simulink model "LETS_GOOOOOO"  (R2020b)
settings: Solver=VariableStepAuto  StartTime=0.0  StopTime=60  RelTol=1e-3
values from neighbouring files (symbols this model uses):
  A_2 = zeros(3)    [MPC_tune.m]
  B_2 = I_inv    [MPC_tune.m]
  C_2 = eye(3)    [MPC_tune.m]
  D_2 = zeros(3)    [MPC_tune.m]
  I_inv = inv(I_mat)    [MPC_tune.m]
  m = 941.102    [Linear_tuning.m]
  TcgCatia = [1 0 0 ... (first row only)    [MPC_tune.m]
undefined symbols (not defined in the file or in its folder): A_kal, B_kal, C_kal, Continuous, D_kal, delta_time, F_tot_max, Fb1_l, Fb1_u, Fb2_l, Fb2_u, Fb3_l, Fb3_u, Fb4_l, Fb4_u, Fc1_l, Fc1_u, Fc2_l, Fc2_u, Fc3_l, Fc3_u, fprop, Ft1_l, Ft1_u, Ft2_l, Ft2_u, Ft3_l, Ft3_u, Ft4_l, Ft4_u, g, r_0, r_cgCatia, r_trajectory, rho, T, t_finalgust, theta0, time, Time, time_delay, Tzy_Shard, u0_final, u0_ini, u1_final, u1_ini, u2_final, u2_ini, u_0, u_1, u_2, v_0, ZI_Cx, ZI_Cy, ZI_Cz, ZI_p, ZI_q, ZI_r
libraries: dspsigops x11, simulink x6, pid_lib x6, fuzblock x3, sharedutil x1, mpclib x1, dspmathops x1, ctrlSharedLib x1
(part 2 of 2)

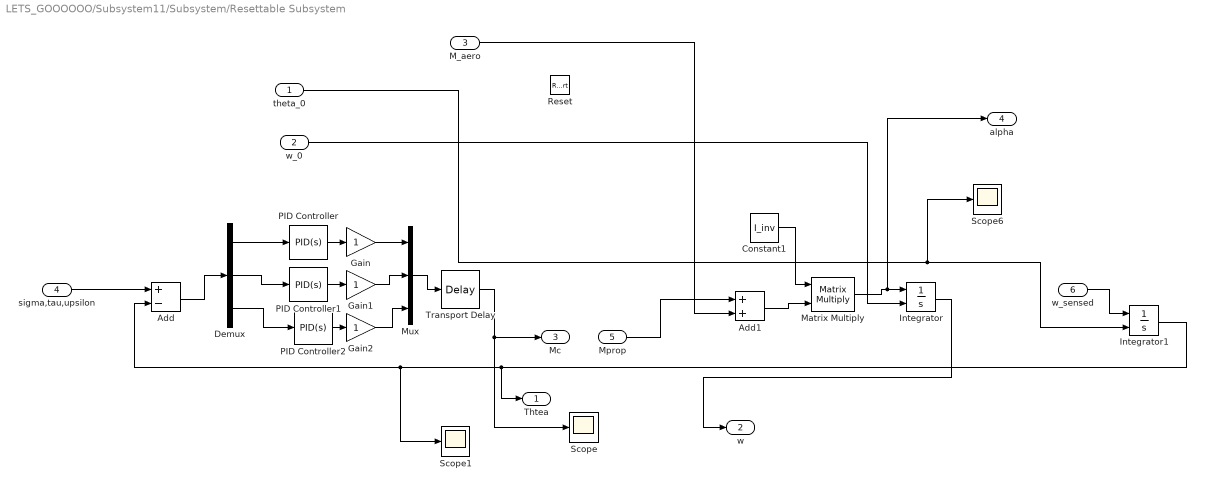
== system LETS_GOOOOOO/Subsystem11/Subsystem/Resettable Subsystem ==
  theta_0 : Inport
  w_0 : Inport  Port=2
  M_aero : Inport  Port=3
  sigma,tau,upsilon : Inport  Port=4
  Mprop : Inport  Port=5
  w_sensed : Inport  Port=6
  Reset : ResetPort  DisableCoverage=on  ResetTriggerType=either
  Add : Sum  Inputs=+-
  Add1 : Sum
  Constant1 : Constant  Value=I_inv
  Demux : Demux  Outputs=3
  Gain : Gain
  Gain1 : Gain
  Gain2 : Gain
  Integrator : Integrator  InitialConditionSource=external  InitialCondition=[0.15;-0.2;0.01]
  Integrator1 : Integrator  InitialConditionSource=external  InitialCondition=[0.01;-0.01;0.005]
  Matrix Multiply : Product  Multiplication=Matrix(*)
  Mux : Mux  Inputs=3
  PID Controller : pid_lib/PID Controller  Controller=PID  Form=Parallel  TimeDomain=Continuous-time  UseExternalTs=off  SampleTime=-1  IntegratorMethod=Forward Euler  FilterMethod=Forward Euler  ControllerParametersSource=internal  P=76.4274415550338  I=3.57793373088927  D=400.875615235633  UseFilter=on  N=5.45397025421619  TunerSelectOption=Transfer Function Based (PID Tuner App)  InitialConditionSource=internal  InitialConditionForIntegrator=0  InitialConditionForFilter=0  DifferentiatorICPrevScaledInput=0  ExternalReset=none  TrackingMode=off  Kt=1  LimitOutput=off  SatLimitsSource=internal  UpperSaturationLimit=inf  LowerSaturationLimit=-inf  LinearizeAsGain=on  AntiWindupMode=none  Kb=1  POutMin=[]  POutMax=[]  IOutMin=[]  IOutMax=[]  DOutMin=[]  DOutMax=[]  NOutMin=[]  NOutMax=[]  SumOutMin=[]  SumOutMax=[]  SaturationOutMin=[]  SaturationOutMax=[]  PParamMin=[]  PParamMax=[]  IParamMin=[]  IParamMax=[]  DParamMin=[]  DParamMax=[]  NParamMin=[]  NParamMax=[]  KbParamMin=[]  KbParamMax=[]  KtParamMin=[]  KtParamMax=[]  KbOutMin=[]  KbOutMax=[]  KtOutMin=[]  KtOutMax=[]  IntegratorOutMin=[]  IntegratorOutMax=[]  FilterOutMin=[]  FilterOutMax=[]  SumI1OutMin=[]  SumI1OutMax=[]  SumI2OutMin=[]  SumI2OutMax=[]  SumI3OutMin=[]  SumI3OutMax=[]  SumI4OutMin=[]  SumI4OutMax=[]  SumDOutMin=[]  SumDOutMax=[]  DifferentiatorOutMin=[]  DifferentiatorOutMax=[]  FilterDiffOutCoefMin=[]  FilterDiffOutCoefMax=[]  ReciprocalOutMin=[]  ReciprocalOutMax=[]  SumDenOutMin=[]  SumDenOutMax=[]  SumNumOutMin=[]  SumNumOutMax=[]  DivideOutMin=[]  DivideOutMax=[]  UdiffTsProdOutMin=[]  UdiffTsProdOutMax=[]  NTsProdOutMin=[]  NTsProdOutMax=[]  UintegralTsProdOutMin=[]  UintegralTsProdOutMax=[]  UngainTsProdOutMin=[]  UngainTsProdOutMax=[]  IntegratorContinuousStateAttributes=''  IntegratorStateMustResolveToSignalObject=off  IntegratorRTWStateStorageClass=Auto  FilterContinuousStateAttributes=''  FilterStateMustResolveToSignalObject=off  FilterRTWStateStorageClass=Auto  ParallelPVariant=InternalParameters  IdealPVariant=Disabled  IVariant=InternalParameters  DVariant=InternalParameters  IntegratorVariant=Continuous  SatVariant=Disabled  AWVariant=Passthrough  PCopyVariant=Disabled  TRVariant=Disabled  FdbkBlocksVariant=Forward  IdealPFdbkVariant=Disabled  SatFdbkVariant=Disabled  DerivativeFilterVariant=ContFilter  NVariant=InternalParameters  NCopyVariant=Disabled  FilterICVariant=InternalICsFilter  IntegratorICVariant=InternalICs  ExternalResetVariant=Disabled  TRSumVariant=Passthrough  SumFdbkVariant=Disabled  SumVariant=Sum_PID  TsampFilterVariant=InternalTs  TsampNgainVariant=Passthrough  TsampIntegralVariant=Passthrough  ExternalSaturationOutDataTypeStr=Inherit: Same as second input
  PID Controller1 : pid_lib/PID Controller  Controller=PID  Form=Parallel  TimeDomain=Continuous-time  UseExternalTs=off  SampleTime=-1  IntegratorMethod=Forward Euler  FilterMethod=Forward Euler  ControllerParametersSource=internal  P=-202.527799620363  I=-9.48129403471772  D=-1062.29457146841  UseFilter=on  N=5.45397025421619  TunerSelectOption=Transfer Function Based (PID Tuner App)  InitialConditionSource=internal  InitialConditionForIntegrator=0  InitialConditionForFilter=0  DifferentiatorICPrevScaledInput=0  ExternalReset=none  TrackingMode=off  Kt=1  LimitOutput=off  SatLimitsSource=internal  UpperSaturationLimit=inf  LowerSaturationLimit=-inf  LinearizeAsGain=on  AntiWindupMode=none  Kb=1  POutMin=[]  POutMax=[]  IOutMin=[]  IOutMax=[]  DOutMin=[]  DOutMax=[]  NOutMin=[]  NOutMax=[]  SumOutMin=[]  SumOutMax=[]  SaturationOutMin=[]  SaturationOutMax=[]  PParamMin=[]  PParamMax=[]  IParamMin=[]  IParamMax=[]  DParamMin=[]  DParamMax=[]  NParamMin=[]  NParamMax=[]  KbParamMin=[]  KbParamMax=[]  KtParamMin=[]  KtParamMax=[]  KbOutMin=[]  KbOutMax=[]  KtOutMin=[]  KtOutMax=[]  IntegratorOutMin=[]  IntegratorOutMax=[]  FilterOutMin=[]  FilterOutMax=[]  SumI1OutMin=[]  SumI1OutMax=[]  SumI2OutMin=[]  SumI2OutMax=[]  SumI3OutMin=[]  SumI3OutMax=[]  SumI4OutMin=[]  SumI4OutMax=[]  SumDOutMin=[]  SumDOutMax=[]  DifferentiatorOutMin=[]  DifferentiatorOutMax=[]  FilterDiffOutCoefMin=[]  FilterDiffOutCoefMax=[]  ReciprocalOutMin=[]  ReciprocalOutMax=[]  SumDenOutMin=[]  SumDenOutMax=[]  SumNumOutMin=[]  SumNumOutMax=[]  DivideOutMin=[]  DivideOutMax=[]  UdiffTsProdOutMin=[]  UdiffTsProdOutMax=[]  NTsProdOutMin=[]  NTsProdOutMax=[]  UintegralTsProdOutMin=[]  UintegralTsProdOutMax=[]  UngainTsProdOutMin=[]  UngainTsProdOutMax=[]  IntegratorContinuousStateAttributes=''  IntegratorStateMustResolveToSignalObject=off  IntegratorRTWStateStorageClass=Auto  FilterContinuousStateAttributes=''  FilterStateMustResolveToSignalObject=off  FilterRTWStateStorageClass=Auto  ParallelPVariant=InternalParameters  IdealPVariant=Disabled  IVariant=InternalParameters  DVariant=InternalParameters  IntegratorVariant=Continuous  SatVariant=Disabled  AWVariant=Passthrough  PCopyVariant=Disabled  TRVariant=Disabled  FdbkBlocksVariant=Forward  IdealPFdbkVariant=Disabled  SatFdbkVariant=Disabled  DerivativeFilterVariant=ContFilter  NVariant=InternalParameters  NCopyVariant=Disabled  FilterICVariant=InternalICsFilter  IntegratorICVariant=InternalICs  ExternalResetVariant=Disabled  TRSumVariant=Passthrough  SumFdbkVariant=Disabled  SumVariant=Sum_PID  TsampFilterVariant=InternalTs  TsampNgainVariant=Passthrough  TsampIntegralVariant=Passthrough  ExternalSaturationOutDataTypeStr=Inherit: Same as second input
  PID Controller2 : pid_lib/PID Controller  Controller=PID  Form=Parallel  TimeDomain=Continuous-time  UseExternalTs=off  SampleTime=-1  IntegratorMethod=Forward Euler  FilterMethod=Forward Euler  ControllerParametersSource=internal  P=-232.294042315359  I=-10.8747940867059  D=-1218.42384402842  UseFilter=on  N=5.45397025421619  TunerSelectOption=Transfer Function Based (PID Tuner App)  InitialConditionSource=internal  InitialConditionForIntegrator=0  InitialConditionForFilter=0  DifferentiatorICPrevScaledInput=0  ExternalReset=none  TrackingMode=off  Kt=1  LimitOutput=off  SatLimitsSource=internal  UpperSaturationLimit=inf  LowerSaturationLimit=-inf  LinearizeAsGain=on  AntiWindupMode=none  Kb=1  POutMin=[]  POutMax=[]  IOutMin=[]  IOutMax=[]  DOutMin=[]  DOutMax=[]  NOutMin=[]  NOutMax=[]  SumOutMin=[]  SumOutMax=[]  SaturationOutMin=[]  SaturationOutMax=[]  PParamMin=[]  PParamMax=[]  IParamMin=[]  IParamMax=[]  DParamMin=[]  DParamMax=[]  NParamMin=[]  NParamMax=[]  KbParamMin=[]  KbParamMax=[]  KtParamMin=[]  KtParamMax=[]  KbOutMin=[]  KbOutMax=[]  KtOutMin=[]  KtOutMax=[]  IntegratorOutMin=[]  IntegratorOutMax=[]  FilterOutMin=[]  FilterOutMax=[]  SumI1OutMin=[]  SumI1OutMax=[]  SumI2OutMin=[]  SumI2OutMax=[]  SumI3OutMin=[]  SumI3OutMax=[]  SumI4OutMin=[]  SumI4OutMax=[]  SumDOutMin=[]  SumDOutMax=[]  DifferentiatorOutMin=[]  DifferentiatorOutMax=[]  FilterDiffOutCoefMin=[]  FilterDiffOutCoefMax=[]  ReciprocalOutMin=[]  ReciprocalOutMax=[]  SumDenOutMin=[]  SumDenOutMax=[]  SumNumOutMin=[]  SumNumOutMax=[]  DivideOutMin=[]  DivideOutMax=[]  UdiffTsProdOutMin=[]  UdiffTsProdOutMax=[]  NTsProdOutMin=[]  NTsProdOutMax=[]  UintegralTsProdOutMin=[]  UintegralTsProdOutMax=[]  UngainTsProdOutMin=[]  UngainTsProdOutMax=[]  IntegratorContinuousStateAttributes=''  IntegratorStateMustResolveToSignalObject=off  IntegratorRTWStateStorageClass=Auto  FilterContinuousStateAttributes=''  FilterStateMustResolveToSignalObject=off  FilterRTWStateStorageClass=Auto  ParallelPVariant=InternalParameters  IdealPVariant=Disabled  IVariant=InternalParameters  DVariant=InternalParameters  IntegratorVariant=Continuous  SatVariant=Disabled  AWVariant=Passthrough  PCopyVariant=Disabled  TRVariant=Disabled  FdbkBlocksVariant=Forward  IdealPFdbkVariant=Disabled  SatFdbkVariant=Disabled  DerivativeFilterVariant=ContFilter  NVariant=InternalParameters  NCopyVariant=Disabled  FilterICVariant=InternalICsFilter  IntegratorICVariant=InternalICs  ExternalResetVariant=Disabled  TRSumVariant=Passthrough  SumFdbkVariant=Disabled  SumVariant=Sum_PID  TsampFilterVariant=InternalTs  TsampNgainVariant=Passthrough  TsampIntegralVariant=Passthrough  ExternalSaturationOutDataTypeStr=Inherit: Same as second input
  Scope : Scope
  Scope1 : Scope
  Scope6 : Scope
  Transport Delay : TransportDelay  DelayTime=0.1
  Thtea : Outport
  w : Outport  Port=2
  Mc : Outport  Port=3
  alpha : Outport  Port=4
  wires:
  Transport Delay/1 -> Mc/1, Scope/1
  Constant1/1 -> Matrix Multiply/1
  PID Controller2/1 -> Gain2/1
  PID Controller/1 -> Gain/1
  Matrix Multiply/1 -> alpha/1, Integrator/1
  Demux/3 -> PID Controller2/1
  Mux/1 -> Transport Delay/1
  sigma,tau,upsilon/1 -> Add/1
  Gain/1 -> Mux/1
  w_0/1 -> Integrator/2
  Gain2/1 -> Mux/3
  Add/1 -> Demux/1
  Add1/1 -> Matrix Multiply/2
  PID Controller1/1 -> Gain1/1
  Integrator/1 -> w/1
  theta_0/1 -> Integrator1/2, Scope6/1
  Demux/2 -> PID Controller1/1
  Gain1/1 -> Mux/2
  M_aero/1 -> Add1/2
  Demux/1 -> PID Controller/1
  Integrator1/1 -> Thtea/1, Scope1/1, Add/2
  Mprop/1 -> Add1/1
  w_sensed/1 -> Integrator1/1

== system LETS_GOOOOOO/Subsystem11/Subsystem/Resettable Subsystem1 ==
  sigma,tau,upsilon : Inport
  Maero : Inport  Port=2
  w0 : Inport  Port=3
  theta0 : Inport  Port=4
  reset : Inport  Port=5
  Mprop : Inport  Port=6
  wsensed : Inport  Port=7
  Add : Sum  Inputs=-+
  Subsystem : Subsystem
  error : Outport
  theta : Outport  Port=2
  w : Outport  Port=3
  Mc : Outport  Port=4
  alpha : Outport  Port=5
  wires:
  theta0/1 -> Subsystem/4(tehat0)
  Subsystem/2(w) -> w/1
  Add/1 -> error/1
  Maero/1 -> Subsystem/1(M_aero)
  sigma,tau,upsilon/1 -> Add/2, Subsystem/2(sigma,tau,upsilon)  "sigma, tau, upsilon"
  Subsystem/1(theta) -> Add/1, theta/1
  w0/1 -> Subsystem/3(w0)
  reset/1 -> Subsystem/5(reset)
  Subsystem/3(Mc) -> Mc/1
  Mprop/1 -> Subsystem/6(Mprop)
  Subsystem/4(alpha) -> alpha/1
  wsensed/1 -> Subsystem/7(wsensed)

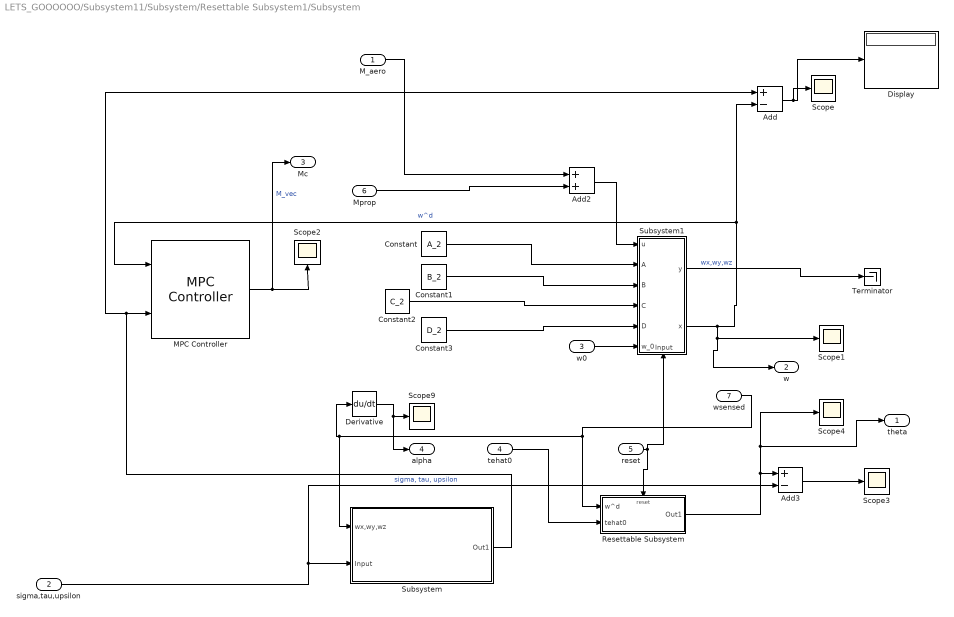
== system LETS_GOOOOOO/Subsystem11/Subsystem/Resettable Subsystem1/Subsystem ==
  M_aero : Inport
  sigma,tau,upsilon : Inport  Port=2
  w0 : Inport  Port=3
  tehat0 : Inport  Port=4
  reset : Inport  Port=5
  Mprop : Inport  Port=6
  wsensed : Inport  Port=7
  Add : Sum  Inputs=+-
  Add2 : Sum
  Add3 : Sum  Inputs=+-
  Constant : Constant  Value=A_2
  Constant1 : Constant  Value=B_2
  Constant2 : Constant  Value=C_2
  Constant3 : Constant  Value=D_2
  Derivative : Derivative
  Display : Display
  MPC Controller : mpclib/MPC Controller  SCDEnableBlockLinearizationSpecification=on  mpcobj=MPCDesignerSession.AppData.Controllers.MPC  is_multiple=0  enable_value=0  return_u0=off  updateMPCinCallerWorkspace=on  md_inport=off  mv_inport=off  uref_inport=off  return_cost=off  return_mvseq=off  return_qpstatus=off  return_xseq=off  return_state=off  return_ovseq=off  state_inport=off  umin_inport=off  umax_inport=off  ymin_inport=off  ymax_inport=off  cc_inport=off  ywt_inport=off  uwt_inport=off  duwt_inport=off  rhoeps_inport=off  pm_inport=off  MaximumP=10  HorizonChoice=FixedHorizon  n_ts=0.1  n_p=10  n_mv=3  n_md=0  n_ud=0  n_mo=3  n_uo=0  BlockDataType=double  SampleTimeInherited=off  switch_inport=off
  Resettable Subsystem : Subsystem  TreatAsAtomicUnit=on
  Scope{,1..4,9} (6 alike) : Scope
  Subsystem : Subsystem
  Subsystem1 : Subsystem
      settings: PortSchema="{\"entries\":[{\"content\":{\"sides\":[{\"content\":{\"connectorIds\":[\"In1\",\"In2\",\"In3\",\"In4\",\"In5\",\"In6\"]},\"type\":\"ConnectorPlacement.EquallySpacedRectSide\",\"uuid\":\"7d9460a7-3adf-4f89-91e7-b456f7078c86\"},{\"content\":{\"connectorIds\":[\"Out1\",\"Out2\"],\"side\":\"RIGHT\"},\"type\":\"ConnectorPlacement.EquallySpacedRectSide\",\"uuid\":\"f1bf29ac-ed67-4ce4-91e2-85f2b90efa08\"},{\"content\":{\"connectorIds\":[],\"side\":\"TOP\"},\"type\":\"ConnectorPlacement.EquallySpacedRectSide\",\"uuid\":\"d922c634-a6d8-424b-a167-3b858780e5fe\"},{\"content\":{\"connectorIds\":[\"In7\"],\"side\":\"BOTTOM\"},\"type\":\"ConnectorPlacement.EquallySpacedRectSide\",\"uuid\":\"f177f641-1570-409d-a38e-cef2b78f705f\"},{\"content\":{\"connectorIds\":[],\"side\":\"HIDDEN\"},\"type\":\"ConnectorPlacement.EquallySpacedRectSide\",\"uuid\":\"30cf80c6-7b26-40df-a778-919a6a544dd2\"}]},\"type\":\"ConnectorPlacement.EquallySpacedConnector\",\"uuid\":\"27252b95-3211-4624-87a6-4be9d32d6c6a\"}],\"packageUris\":[\"http://schema.mathworks.com/mf0/Connector/R2020b\"],\"version\":\"1.0\"}"
  Terminator : Terminator
  theta : Outport
  w : Outport  Port=2
  Mc : Outport  Port=3
  alpha : Outport  Port=4
  wires:
  Subsystem1/1(y) -> Terminator/1  "wx,wy,wz"
  Derivative/1 -> alpha/1, Scope9/1
  Resettable Subsystem/1(Out1) -> Scope4/1, theta/1, Add3/1
  Add/1 -> Display/1, Scope/1
  Add3/1 -> Scope3/1
  Add2/1 -> Subsystem1/1(u)
  sigma,tau,upsilon/1 -> Add3/2, Subsystem/2(Input)  "sigma, tau, upsilon"
  Subsystem/1(Out1) -> Add/1, MPC Controller/2
  M_aero/1 -> Add2/1
  Constant2/1 -> Subsystem1/4(C)
  Constant3/1 -> Subsystem1/5(D)
  Subsystem1/2(x) -> Add/2, MPC Controller/1, w/1, Scope1/1  "w^d"
  MPC Controller/1 -> Mc/1, Scope2/1  "M_vec"
  Constant/1 -> Subsystem1/2(A)
  Constant1/1 -> Subsystem1/3(B)
  w0/1 -> Subsystem1/6(w_0)
  tehat0/1 -> Resettable Subsystem/2(tehat0)
  reset/1 -> Subsystem1/7(Input), Resettable Subsystem/Reset
  Mprop/1 -> Add2/2
  wsensed/1 -> Resettable Subsystem/1(w^d), Subsystem/1(wx,wy,wz), Derivative/1

== system LETS_GOOOOOO/Subsystem11/Subsystem/Resettable Subsystem1/Subsystem/Resettable Subsystem ==
  w^d : Inport
  tehat0 : Inport  Port=2
  Reset : ResetPort  DisableCoverage=on
  Integrator : Integrator  InitialConditionSource=external  InitialCondition=theta0
  Scope : Scope
  Out1 : Outport
  wires:
  tehat0/1 -> Integrator/2
  w^d/1 -> Integrator/1
  Integrator/1 -> Scope/1, Out1/1

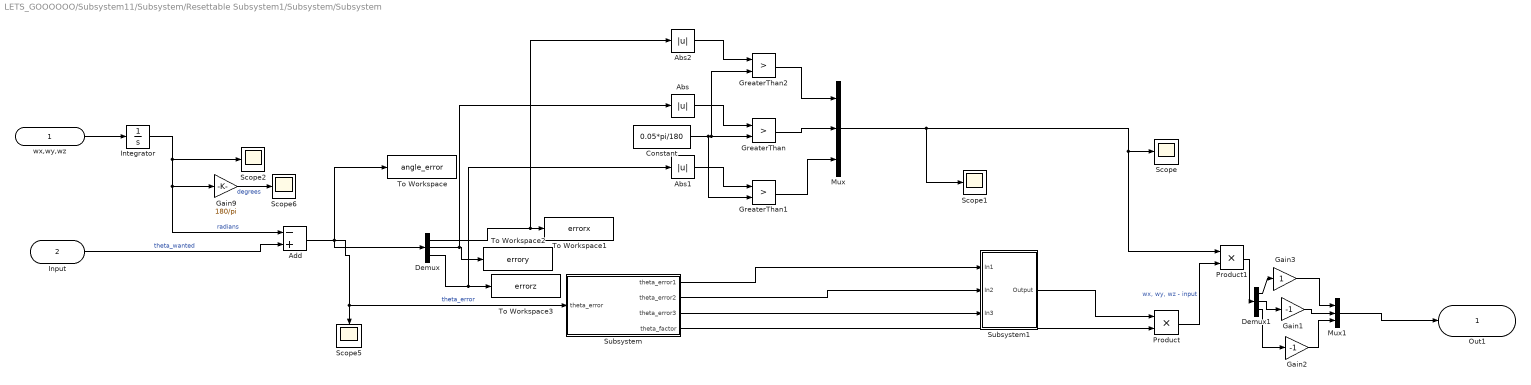
== system LETS_GOOOOOO/Subsystem11/Subsystem/Resettable Subsystem1/Subsystem/Subsystem ==
  wx,wy,wz : Inport
  Input : Inport  Port=2
  Abs : Abs
  Abs1 : Abs
  Abs2 : Abs
  Add : Sum  Inputs=-+
  Constant : Constant  Value=0.05*pi/180
  Demux : Demux  Outputs=3
  Demux1 : Demux  Outputs=3
  Gain1 : Gain  Gain=-1
  Gain2 : Gain  Gain=-1
  Gain3 : Gain
  Gain9 : Gain  Gain=180/pi
  GreaterThan : RelationalOperator  Operator=>  OutDataTypeStr=boolean  RndMeth=Simplest
  GreaterThan1 : RelationalOperator  Operator=>  OutDataTypeStr=boolean  RndMeth=Simplest
  GreaterThan2 : RelationalOperator  Operator=>  OutDataTypeStr=boolean  RndMeth=Simplest
  Integrator : Integrator  InitialCondition=[0;0;0]
  Mux : Mux  Inputs=3
  Mux1 : Mux  Inputs=3
  Product : Product
  Product1 : Product
  Scope{,1..2,5..6} (5 alike) : Scope
  Subsystem : Subsystem
  Subsystem1 : Subsystem
  To Workspace : ToWorkspace  VariableName=angle_error  SampleTime=-1
  To Workspace1 : ToWorkspace  VariableName=errorx  SaveFormat=Timeseries  SampleTime=-1
      settings: Save2DSignal=2-D array (concatenate along first dimension)
  To Workspace2 : ToWorkspace  VariableName=errory  SaveFormat=Timeseries  SampleTime=-1
  To Workspace3 : ToWorkspace  VariableName=errorz  SaveFormat=Timeseries  SampleTime=-1
  Out1 : Outport
  wires:
  Integrator/1 -> Add/1, Gain9/1, Scope2/1  "radians"
  Add/1 -> To Workspace/1, Demux/1, Subsystem/1(theta_error), Scope5/1  "theta_error"
  Gain9/1 -> Scope6/1  "degrees"
  Input/1 -> Add/2  "theta_wanted"
  Product/1 -> Product1/2  "wx, wy, wz - input"
  wx,wy,wz/1 -> Integrator/1
  Subsystem/4(theta_factor) -> Product/2
  Demux/2 -> Abs/1, To Workspace2/1
  Demux/3 -> Abs1/1, To Workspace3/1
  Demux/1 -> Abs2/1, To Workspace1/1
  Subsystem/1(theta_error1) -> Subsystem1/1(In1)
  Subsystem/2(theta_error2) -> Subsystem1/2(In2)
  Subsystem/3(theta_error3) -> Subsystem1/3(In3)
  Subsystem1/1(Output) -> Product/1
  Abs/1 -> GreaterThan/1
  Constant/1 -> GreaterThan1/2, GreaterThan2/2, GreaterThan/2
  Abs1/1 -> GreaterThan1/1
  Abs2/1 -> GreaterThan2/1
  GreaterThan2/1 -> Mux/1
  GreaterThan/1 -> Mux/2
  GreaterThan1/1 -> Mux/3
  Mux/1 -> Scope1/1, Scope/1, Product1/1
  Product1/1 -> Demux1/1
  Mux1/1 -> Out1/1
  Demux1/2 -> Gain1/1
  Demux1/3 -> Gain2/1
  Demux1/1 -> Gain3/1
  Gain3/1 -> Mux1/1
  Gain1/1 -> Mux1/2
  Gain2/1 -> Mux1/3

== system LETS_GOOOOOO/Subsystem11/Subsystem/Resettable Subsystem1/Subsystem/Subsystem1 ==
  u : Inport
  A : Inport  Port=2
  B : Inport  Port=3
  C : Inport  Port=4
  D : Inport  Port=5
  w_0 : Inport  Port=6
  Input : Inport  Port=7
  Product{,1..3} (4 alike) : Product  SCDEnableBlockLinearizationSpecification=on  Multiplication=Matrix(*)
  Resettable Subsystem : Subsystem  TreatAsAtomicUnit=on
  Sum : Sum  Inputs=|++
  Sum1 : Sum  Inputs=++|
  dxTerm : Terminator
  y : Outport  VectorParamsAs1DForOutWhenUnconnected=off
  x : Outport  Port=2  VectorParamsAs1DForOutWhenUnconnected=off
  wires:
  Sum/1 -> Resettable Subsystem/1(alpha), dxTerm/1  "dx"
  Product3/1 -> Sum1/1  "Cx"
  Product/1 -> Sum/1  "Bu"
  u/1 -> Product2/2, Product/2
  Product2/1 -> Sum1/2  "Du"
  Resettable Subsystem/1(x) -> x/1, Product1/2, Product3/2  "x"
  A/1 -> Product1/1
  Product1/1 -> Sum/2  "Ax"
  C/1 -> Product3/1
  B/1 -> Product/1
  D/1 -> Product2/1
  Sum1/1 -> y/1
  w_0/1 -> Resettable Subsystem/2(omega0)
  Input/1 -> Resettable Subsystem/Reset

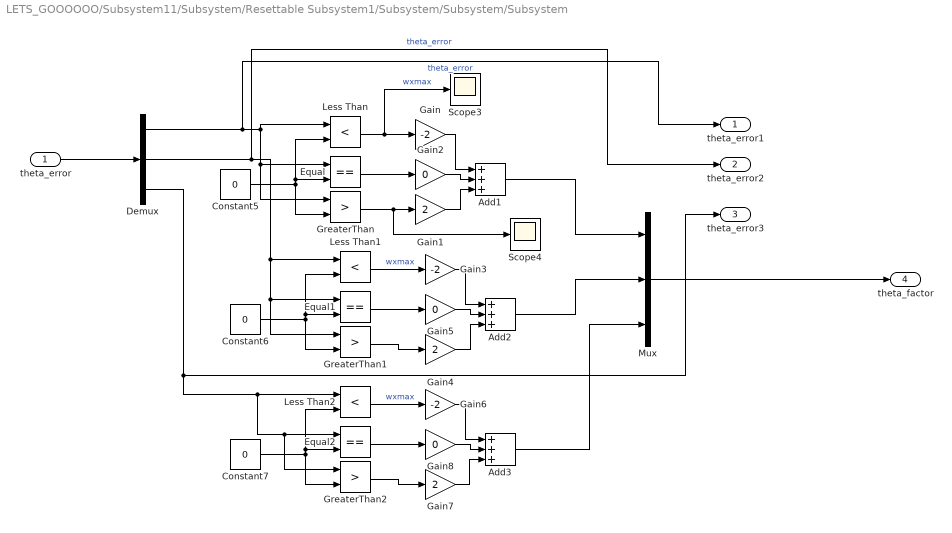
== system LETS_GOOOOOO/Subsystem11/Subsystem/Resettable Subsystem1/Subsystem/Subsystem/Subsystem ==
  theta_error : Inport
  Add1 : Sum  Inputs=+++
  Add2 : Sum  Inputs=+++
  Add3 : Sum  Inputs=+++
  Constant5 : Constant  Value=0
  Constant6 : Constant  Value=0
  Constant7 : Constant  Value=0
  Demux : Demux  Outputs=3
  Equal : RelationalOperator  Operator===  OutDataTypeStr=boolean  RndMeth=Simplest
  Equal1 : RelationalOperator  Operator===  OutDataTypeStr=boolean  RndMeth=Simplest
  Equal2 : RelationalOperator  Operator===  OutDataTypeStr=boolean  RndMeth=Simplest
  Gain : Gain  Gain=-2
  Gain1 : Gain  Gain=2
  Gain2 : Gain  Gain=0
  Gain3 : Gain  Gain=-2
  Gain4 : Gain  Gain=2
  Gain5 : Gain  Gain=0
  Gain6 : Gain  Gain=-2
  Gain7 : Gain  Gain=2
  Gain8 : Gain  Gain=0
  GreaterThan : RelationalOperator  Operator=>  OutDataTypeStr=boolean  RndMeth=Simplest
  GreaterThan1 : RelationalOperator  Operator=>  OutDataTypeStr=boolean  RndMeth=Simplest
  GreaterThan2 : RelationalOperator  Operator=>  OutDataTypeStr=boolean  RndMeth=Simplest
  Less Than : RelationalOperator  Operator=<  OutDataTypeStr=boolean  RndMeth=Simplest
  Less Than1 : RelationalOperator  Operator=<  OutDataTypeStr=boolean  RndMeth=Simplest
  Less Than2 : RelationalOperator  Operator=<  OutDataTypeStr=boolean  RndMeth=Simplest
  Mux : Mux  Inputs=3
  Scope3 : Scope
  Scope4 : Scope
  theta_error1 : Outport
  theta_error2 : Outport  Port=2
  theta_error3 : Outport  Port=3
  theta_factor : Outport  Port=4
  wires:
  Add1/1 -> Mux/1
  Constant5/1 -> Equal/2, Less Than/2, GreaterThan/2
  Equal2/1 -> Gain8/1
  Demux/1 -> theta_error1/1, GreaterThan/1, Equal/1, Less Than/1  "theta_error"
  GreaterThan2/1 -> Gain7/1
  Gain1/1 -> Add1/3
  Gain7/1 -> Add3/3
  Less Than1/1 -> Gain3/1  "wxmax"
  Gain6/1 -> Add3/1
  Equal/1 -> Gain2/1
  Gain5/1 -> Add2/2
  Add3/1 -> Mux/3
  GreaterThan/1 -> Scope4/1, Gain1/1
  Constant6/1 -> Equal1/2, Less Than1/2, GreaterThan1/2
  Demux/3 -> theta_error3/1, GreaterThan2/1, Equal2/1, Less Than2/1
  Gain3/1 -> Add2/1
  Constant7/1 -> Equal2/2, Less Than2/2, GreaterThan2/2
  Equal1/1 -> Gain5/1
  Gain8/1 -> Add3/2
  Gain4/1 -> Add2/3
  GreaterThan1/1 -> Gain4/1
  Gain/1 -> Add1/1
  Demux/2 -> theta_error2/1, GreaterThan1/1, Equal1/1, Less Than1/1  "theta_error"
  Gain2/1 -> Add1/2
  Add2/1 -> Mux/2
  Less Than/1 -> Scope3/1, Gain/1  "wxmax"
  Less Than2/1 -> Gain6/1  "wxmax"
  theta_error/1 -> Demux/1
  Mux/1 -> theta_factor/1

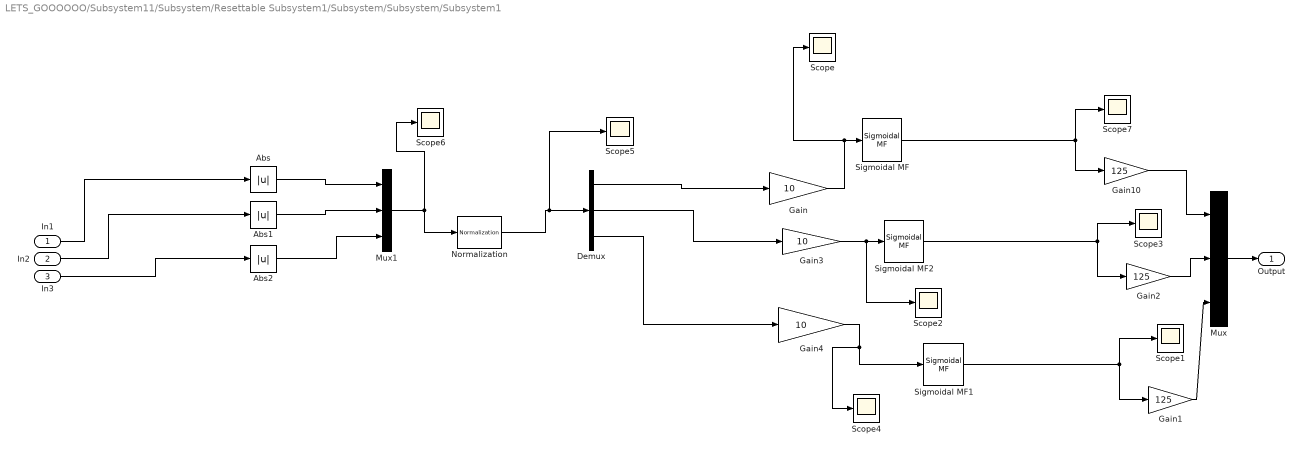
== system LETS_GOOOOOO/Subsystem11/Subsystem/Resettable Subsystem1/Subsystem/Subsystem/Subsystem1 ==
  In1 : Inport
  In2 : Inport  Port=2
  In3 : Inport  Port=3
  Abs : Abs
  Abs1 : Abs
  Abs2 : Abs
  Demux : Demux  Outputs=3
  Gain : Gain  Gain=10
  Gain1 : Gain  Gain=125
  Gain10 : Gain  Gain=125
  Gain2 : Gain  Gain=125
  Gain3 : Gain  Gain=10
  Gain4 : Gain  Gain=10
  Mux : Mux  Inputs=3
  Mux1 : Mux  Inputs=3
  Normalization : dspmathops/Normalization  NormType=Squared 2-norm  Bias=1e-10  NormOver=Each column  Dimension=1  roundingMode=Floor  overflowMode=off  accumDataTypeStr=Inherit: Same as product output  accumLastDataTypeStr=Inherit: Same as product output  outputDataTypeStr=Inherit: Same as product output  outputMin=[]  outputMax=[]  outputLastDataTypeStr=Inherit: Same as product output
  Scope{,1..7} (8 alike) : Scope
  Sigmoidal MF : fuzblock/Membership  Functions/Sigmoidal MF  a=10^(-8)  c=1000
      settings: SourceProductBaseCode=FL
  Sigmoidal MF1 : fuzblock/Membership  Functions/Sigmoidal MF  a=10^(-8)  c=1000
      settings: SourceProductBaseCode=FL
  Sigmoidal MF2 : fuzblock/Membership  Functions/Sigmoidal MF  a=10^(-8)  c=1000
      settings: SourceProductBaseCode=FL
  Output : Outport
  wires:
  Gain2/1 -> Mux/2
  Gain10/1 -> Mux/1
  Sigmoidal MF1/1 -> Gain1/1, Scope1/1
  Sigmoidal MF/1 -> Gain10/1, Scope7/1
  Sigmoidal MF2/1 -> Gain2/1, Scope3/1
  Gain/1 -> Scope/1, Sigmoidal MF/1
  Gain1/1 -> Mux/3
  Gain3/1 -> Scope2/1, Sigmoidal MF2/1
  In2/1 -> Abs1/1
  In1/1 -> Abs/1
  In3/1 -> Abs2/1
  Mux/1 -> Output/1
  Abs/1 -> Mux1/1
  Abs1/1 -> Mux1/2
  Gain4/1 -> Scope4/1, Sigmoidal MF1/1
  Abs2/1 -> Mux1/3
  Demux/3 -> Gain4/1
  Demux/1 -> Gain/1
  Demux/2 -> Gain3/1
  Mux1/1 -> Normalization/1, Scope6/1
  Normalization/1 -> Scope5/1, Demux/1

== system LETS_GOOOOOO/Subsystem11/Subsystem/Resettable Subsystem1/Subsystem/Subsystem1/Resettable Subsystem ==
  alpha : Inport
  omega0 : Inport  Port=2
  Reset : ResetPort  DisableCoverage=on
  Integrator : Integrator  InitialConditionSource=external  InitialCondition=theta0
  Scope : Scope
  x : Outport
  wires:
  omega0/1 -> Integrator/2
  alpha/1 -> Integrator/1
  Integrator/1 -> Scope/1, x/1

== matlab function LETS_GOOOOOO/Subsystem5/Subsystem/MATLAB Function6 ==
  data: F_y input; F_c1 output; M_x input; M_z input; F_c2 output; F_c3 output
function [F_c1, F_c2, F_c3] = fcn(F_y, M_x, M_z)
%CATIA trans
TcgCatia = [1 0 0;
    0 -1 0;
    0 0 -1];

%Propeller arms - changed due to CATIA errors
c_1 = [-640.1998; 0; 506.566]*10^(-3);      %Control Back Top
c_2 = [-1040.1998; 0; -493.434]*10^(-3);    %Control Back Bottom
c_3 = [2259.8002; 0; -293.434]*10^(-3);     %Control Front

%Propeller arms - rotated
c_1 = TcgCatia*c_1;
c1 = transpose(c_1);
c_2 = TcgCatia*c_2;
c2 = transpose(c_2);
c_3 = TcgCatia*c_3;
c3 = transpose(c_3);

xc_1 = c1(1);
zc_1 = c1(3);

xc_2 = c2(1);
zc_2 = c2(3);

xc_3 = c3(1);
zc_3 = c3(3);

A_control = [1 1 1;
    zc_1 zc_2 zc_3;
    xc_1 xc_2 xc_3];
A_cinv = inv(A_control);
force_control = [F_y; M_x; M_z];
controlvec = A_cinv*force_control;
F_c1 = controlvec(1);
F_c2 = controlvec(2);
F_c3 = controlvec(3);
end

== matlab function LETS_GOOOOOO/Subsystem5/MATLAB Function4 ==
  data: F1 input; F_t1 output; F2 input; F3 input; F_t2 output; F_t3 output; F_t4 output; F_b1 output; F_b2 output; F_b3 output; F_b4 output
function [F_t1, F_t2, F_t3, F_t4, F_b1, F_b2, F_b3, F_b4] = fcn(F1, F2, F3)
%F3 is one prop
%F1 is two props
%F2 is two props
F_t1 = F1/2;
F_t2 = F_t1;
F_t3 = F3;
F_t4 = F_t3;
F_b3 = F_t3;
F_b4 = F_t3;
F_b1 = F2/2;
F_b2 = F_b1;

Ft = [F_t1, F_t2, F_t3, F_t4];
Fb = [F_b1, F_b2, F_b3, F_b4];
end

== matlab function LETS_GOOOOOO/Subsystem5/Subsystem3/MATLAB Function7 ==
  data: F1 input; F_z output; F2 input; M_y output; F3 input
function [F_z, M_y] = fcn(F1, F2, F3)
xt_1 = 1.2598;
xb_1 = 2.2598;
xt_3 = -1.3402;
x_t1 = xt_1;
x_b1 = xb_1;
x_t3 = xt_3;

M_y = -100;
F_z = 0;

A_mat = [1 1;
    xt_1 xb_1];

A_inv = inv(A_mat);

force = [F1; F2];

back = A_mat*force;
backtrack = [4*F3; 4*F3*xt_3];
forceback = back+backtrack;
F_z = forceback(1);
M_y = forceback(2) + 0.15;
end

== matlab function LETS_GOOOOOO/Subsystem5/Subsystem3/MATLAB Function8 ==
  data: F_c1 input; F_y output; M_x output; F_c2 input; F_c3 input; M_z output
function [F_y, M_x, M_z] = fcn(F_c1, F_c2, F_c3)

%CATIA trans
TcgCatia = [1 0 0;
    0 -1 0;
    0 0 -1];

%Propeller arms - changed due to CATIA errors
c_1 = [-640.1998; 0; 506.566]*10^(-3);      %Control Back Top
c_2 = [-1040.1998; 0; -493.434]*10^(-3);    %Control Back Bottom
c_3 = [2259.8002; 0; -293.434]*10^(-3);     %Control Front

%Propeller arms - rotated
c_1 = TcgCatia*c_1;
c1 = transpose(c_1);
c_2 = TcgCatia*c_2;
c2 = transpose(c_2);
c_3 = TcgCatia*c_3;
c3 = transpose(c_3);

xc_1 = c1(1);
zc_1 = c1(3);

xc_2 = c2(1);
zc_2 = c2(3);

xc_3 = c3(1);
zc_3 = c3(3);


Control_forces = [F_c1; F_c2; F_c3];

A_control = [1 1 1;
        zc_1 zc_2 zc_3;
        xc_1 xc_2 xc_3]; 
Control_vec_2 = A_control*Control_forces;
F_y = Control_vec_2(1);
M_x = Control_vec_2(2);
M_z = Control_vec_2(3);
end

== matlab function LETS_GOOOOOO/Subsystem5/Subsystem3/MATLAB Function9 ==
  data: Ft1 input; F1 output; Ft2 input; F2 output; F3 output; Ft3 input; Ft4 input; Fb1 input; Fb2 input; Fb3 input; Fb4 input
function [F1, F2, F3] = fcn(Ft1, Ft2, Ft3, Ft4, Fb1, Fb2, Fb3, Fb4)
%F3 is one prop
%F1 is two props
%F2 is two props
F1 = 2*Ft1;
F2 = 2*Fb1;
F3 = Ft3;
end

== matlab function LETS_GOOOOOO/Subsystem4/MATLAB Function2 ==
  data: theta_x input; Transformation_Mat output; theta_y input; theta_z input
function Transformation_Mat  = Euler(theta_x, theta_y, theta_z)

a = cos(theta_x)*cos(theta_z);
b = cos(theta_x)*sin(theta_z);
c = - sin(theta_x);
d = sin(theta_y)*sin(theta_x)*cos(theta_z) - cos(theta_y)*sin(theta_z);
e = sin(theta_y)*sin(theta_x)*sin(theta_z) + cos(theta_y)*cos(theta_z);
f = sin(theta_y)*cos(theta_x);
g = cos(theta_y)*sin(theta_x)*cos(theta_z) + sin(theta_y)*sin(theta_z);
h = cos(theta_y)*sin(theta_x)*sin(theta_z) - sin(theta_y)*cos(theta_z);
i = cos(theta_y)*cos(theta_x);

Transformation_Mat = [a b c;
    d e f;
    g h i];


end

== matlab function LETS_GOOOOOO/Subsystem9/GPS Model ==
  settings: updateMethod=DISCRETE
  data: position input; newposition output
function newposition  = gps(position)

    % Input: position
    % Output: position with gps accuracies inclduded
    mu = 0; 
    sigma = 0.015;

    r1 = normrnd(mu, sigma);
    r2 = normrnd(mu, sigma);
    r3 = normrnd(mu, sigma);

    newposition = [0,0,0];

    newposition(1) = position(1) + r1;
    newposition(2) = position(2) + r2;
    newposition(3) = position(3) + r3;

end

== matlab function LETS_GOOOOOO/Subsystem4/MATLAB Function3 ==
  data: theta_x input; Transformation_Mat output; theta_y input; theta_z input
function Transformation_Mat  = Euler(theta_x, theta_y, theta_z)

a = cos(theta_x)*cos(theta_z);
b = cos(theta_x)*sin(theta_z);
c = - sin(theta_x);
d = sin(theta_y)*sin(theta_x)*cos(theta_z) - cos(theta_y)*sin(theta_z);
e = sin(theta_y)*sin(theta_x)*sin(theta_z) + cos(theta_y)*cos(theta_z);
f = sin(theta_y)*cos(theta_x);
g = cos(theta_y)*sin(theta_x)*cos(theta_z) + sin(theta_y)*sin(theta_z);
h = cos(theta_y)*sin(theta_x)*sin(theta_z) - sin(theta_y)*cos(theta_z);
i = cos(theta_y)*cos(theta_x);

Transformation_Mat = [a b c;
    d e f;
    g h i];


end

== matlab function LETS_GOOOOOO/Subsystem5/Subsystem/MATLAB Function ==
  data: My input; Ft1 output; Fz input; Ft2 output; Ft3 output; Ft4 output; Fb1 output; Fb2 output; Fb3 output; Fb4 output
function [Ft1, Ft2, Ft3, Ft4, Fb1, Fb2, Fb3, Fb4] = fixingpropulsionsmess(My, Fz)
xt_1 = 1.2598;
xb_1 = 2.2598;
xt_3 = -1.3402;
xb_3 = -1.3402;
x_t1 = xt_1;
x_b1 = xb_1;
x_t3 = xt_3;
x_b3 = xb_3;;

%alpha_1 = (-2*xt_1*(1/((xt_1/xb_1)-1))*(2 - (2*xb_3/xb_1)) - 4*xb_3)^2;
%alpha_2 = ((1/((xt_1/xb_1)-1))*(2-(2*xb_3/xb_1)))^2;
%alpha = alpha_1 + alpha_2;

%beta_1 = 2*My*((1/(2*xb_1))*(1 - (xt_1/xb_1)*(1/((xt_1/xb_1) -1))));
%beta_2 = 2*My*(1/((xt_1/xb_1) -1))*(1/(2*xb_1))*(1/((xt_1/xb_1) -1))*(2 - ((2*xb_3)/x_b1));
%beta_3 = 2*Fz*(1/(2*xb_1)*xt_1*(1/(xt_1/xb_1 -1)));
%beta_4 = 2*Fz*(-1/2*(1/(xt_1/xb_1 -1))*(1/(xt_1/xb_1 -1))*(2-2*xb_3/xb_1));
%beta = beta_1 + beta_2 + beta_3 + beta_4;

%a = beta/(2*alpha);
%y = 1/(2*xb_1)*(My - 2*xt_1*(1/(xt_1/xb_1 -1))*(-0.5*Fz + 2*(2 - 2*xb_3/xb_1)*a + 1/(2*xb_1)*My) - 4*xb_3*a);
%x = (1/(xt_1/xb_1 -1))*(-0.5*Fz + (2 - 2*xb_3/xb_1)*a + 1/(2*xb_1)*My);

a_num = 2/((2*xb_1 - 2*xt_1)^2) *(2*(4*xt_1 - 4*xb_3)*(My - Fz*0.5)) + 2*Fz + (4*My - Fz*(2 + 4*xt_1 - 4*xb_3))/(2*xb_1 - 2*xt_1);
a_den = -(2/((2*xb_1 - 2*xt_1)^2)*2*((4*xt_1 - 4*xb_3)^2) + 10 + (8*(4*xt_1 - 4*xb_3))/(-2*xt_1 + 2*xb_1));
a = a_num/a_den;

y = 1/(-2*xt_1 + 2*xb_1)*(a*(4*xt_1 - 4*xb_3) + My - 0.5*Fz);
x = -y - 2*a + Fz/2;
z = a;

Ft1 = x;
Ft2 = Ft1;
Ft3 = a;
Ft4 = Ft3;
Fb1 = y;
Fb2 = Fb1;
Fb3 = Ft3;
Fb4 = Ft3;
end

== matlab function LETS_GOOOOOO/Subsystem2/MATLAB Function1 ==
  settings: updateMethod=DISCRETE
  data: angvel input; accelData output; acc input
function accelData = accelerometer(angvel, acc)

    %
    % Create gyroscope sensor object
    params = accelparams;
    
    % Parameters for simulated signal
    N = 1;       % Number of samples
    Fs = 100000;       % Sampling rate
    %Fc = 0.25;      % Sinusoidal frequency
    
    
    % Create arrays
    t = (0:(1/Fs):((N-1)/Fs)).';
    acc = acc;          %Input accelerations
    orient = quaternion.ones(N, 1);
    angvel = angvel;
    
    % Generate acceleration data
    imu = imuSensor('SampleRate', Fs, 'Accelerometer', params);
    imu.Accelerometer.MeasurementRange = 1000;   % Maximum acceleration accelerometer can measure
    imu.Accelerometer.Resolution = 1/Fs;           % Step size of digital measurements
    
    % Biases
    imu.Accelerometer.BiasInstability = 0.000000000001; 7.5 / 1000 * 9.81;
    imu.Accelerometer.NoiseDensity = 0.000000000001;%150 / 1000 / 1000 * 9.81 /10; 
    imu.Accelerometer.TemperatureBias = 50 / 1000 / 1000 * 9.81;
    
  
    
    accelData = imu(acc, angvel, orient);
    
    accelData(:,3) = accelData(:,3) - 9.81;

    accelData(:,1) = accelData(:,1) * -1;
    accelData(:,2) = accelData(:,2) * -1;
    accelData(:,3) = accelData(:,3) * -1;

end

== matlab function LETS_GOOOOOO/Subsystem3/MATLAB Function10 ==
  settings: updateMethod=DISCRETE
  data: xvel input; yvel input; zvel input; wx output; accx input; accy input; accz input; wy output; wz output
function [wx, wy, wz]  = fungyroscope(xvel, yvel, zvel, accx, accy, accz)
   
    % Create gyroscope sensor object
    params = gyroparams;         
    
    % Parameters for simulated signal
    N = 1;       % Number of samples
    Fs = 100;       % Sampling rate
    Fc = 0.25;      % Sinusoidal frequency
    
    % Create arrays
    t = (0:(1/Fs):((N-1)/Fs)).';
    acc = [accx, accy, accz];          % Input accelerations
    angvel = [xvel,yvel,zvel];
    %angvel(:,1) = 8*sin(2*pi*Fc*t);
    
    % Generate gyroscopic data
    imu = imuSensor('SampleRate', Fs, 'Gyroscope', params);
    %imu.Gyroscope.MeasurementRange = 1000;   % Maximum angular velocity gyroscope can measure
    %imu.Gyroscope.Resolution = 1/Fs;           % Step size of digital measurements
    
    % Biases
    
    %imu.Gyroscope.BiasInstability = 0.012 * 3.14159 / 180;       % rad/hr
    %imu.Gyroscope.NoiseDensity = 0.15 * 3.14159 / 180;          % rad/s
    %imu.Gyroscope.RandomWalk = 0.017 * 3.14159 / 180;           % rad/sqrt(hr)
    %imu.Gyroscope.TemperatureBias = 0.25 * 3.14159 / 180;       % rad/s
    %imu.Gyroscope.AccelerationBias = 0.3;
    
    % Define real accelerations
    %acc(:,1) = 1;
    [~, gyroData] = imu(acc, angvel, eye(3));
    
    wx = gyroData(1);
    wy = gyroData(2);
    wz = gyroData(3);

end

== matlab function LETS_GOOOOOO/Subsystem1/MATLAB Function ==
  data: t input; u_0 output; u0 input; u1 input; u2 input; deltat input; u_1 output; u_2 output
function [u_0, u_1, u_2] = fcn(t, u0, u1, u2, deltat)

point = (t+deltat)/deltat;
point = round(point);
if point > length(u0)
    u_0 = u0(length(u0));
    u_1 = u1(length(u1));
    u_2 = u2(length(u2));
else
    u_0 = u0(point);
    u_1 = u1(point);
    u_2 = u2(point);
end

end

== matlab function LETS_GOOOOOO/Subsystem5/MATLAB Function5 ==
  data: M_y input; F1 output; F_z input; F2 output; F3 output
function [F1, F2, F3] = fcn(M_y, F_z)
xt_1 = 1.2598;
xb_1 = 2.2598;
xt_3 = -1.3402;
x_t1 = xt_1;
x_b1 = xb_1;
x_t3 = xt_3;



A_mat = [1 1;
    xt_1 xb_1];

A_inv = inv(A_mat);

p_0 = 0.2;
p_minus1 = 0;
step = 1000;
Converged = 0;
p_list = [];
x_list = [];
y_list = [];
J_list = [];
Fzz =[];
Myy =[];
while Converged == 0
    B = [(F_z - 4*p_0); (M_y - 4*p_0*xt_3)];
    force_0 = (A_inv*B);
    J_0 = sqrt(force_0(1)^2 + force_0(2)^2 + p_0^2);
    back = A_mat*force_0;
    backtrack = [4*p_0; 4*p_0*xt_3];
    forceback = back+backtrack;
    diff = sum(abs(forceback - [F_z; M_y]));
    if diff > 10^(-7)
        disp('Error')
        break
    end
    force = force_0;
    J = J_0;
    p = p_0;
    
    p_1 = p_0 + step;
    B = [(F_z - 4*p_1); (M_y - 4*p_1*xt_3)];
    force_1 = (A_inv*B);
    J_1 = sqrt(force_1(1)^2 + force_1(2)^2 + p_1^2);
    back = A_mat*force_1;
    backtrack = [4*p_1; 4*p_1*xt_3];
    forceback = back+backtrack;
    diff = sum(abs(forceback - [F_z; M_y]));
    if diff > 10^(-7)
        disp('Error')
        break
    end
    if J_1 < J_0
        force = force_1;
        J = J_1;
        p = p_1;
    end
    
    p_2 = p_0 - step;
    B = [(F_z - 4*p_2); (M_y - 4*p_2*xt_3)];
    force_2 = (A_inv*B);
    J_2 = sqrt(force_2(1)^2 + force_2(2)^2 + p_2^2);
    back = A_mat*force_2;
    backtrack = [4*p_2; 4*p_2*xt_3];
    forceback = back+backtrack;
    diff = sum(abs(forceback - [F_z; M_y]));
    if diff > 10^(-7)
        disp('Error')
        break
    end
    if J_2 < J_0 && J_2 < J_1
        force = force_2;
        J = J_2;
        p = p_2;
    end
    
    if p_minus1 < p_0 && p_0 < p
        step = step;
    elseif p_minus1 > p_0 && p_0 > p
        step = step;
    else
        step = step*0.9;
    end
        
    p_minus1 = p_0;
    p_0 = p;
    p_list = [p_list; p_0];
    x_list = [x_list; force(1)];
    y_list = [y_list; force(2)];
    J_list = [J_list; J];
    if step < abs(min([F_z,M_y])*10^(-9))
        Converged = 1;
    end
    
    
end

F1 = x_list(length(x_list));
F2 = y_list(length(y_list));
F3 = p_0;
end
